simulink model "RC_Circuit_N16C_1"  (R2020b)
settings: Solver=VariableStepAuto  StartTime=0.0  StopTime=10.0  RelTol=1e-3
model workspace (MAT data in the model file):
  Cp = 1.49336e-12
  Cs = 9.6952e-12
  L = 1.154625e-06
  R = 24.7254
libraries: powerlib x51
settings Model: OrderedModelArguments=off  Creator=25085  LastModifiedBy=zq001
settings DebuggingCC: UnconnectedLineMsg=none

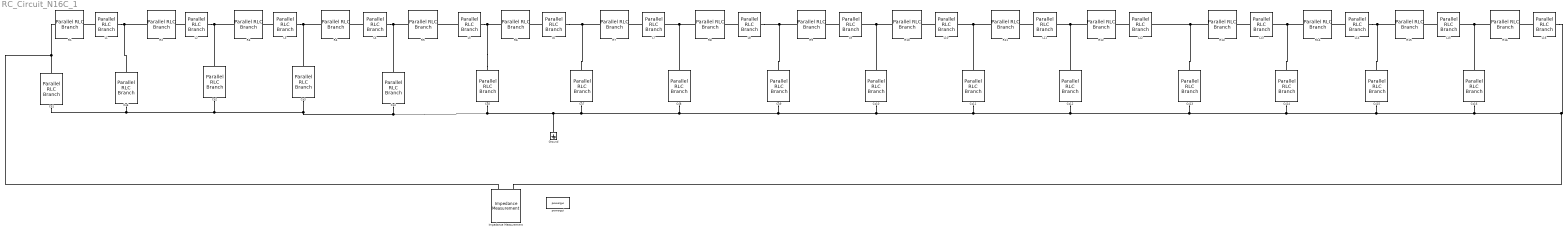
== system RC_Circuit_N16C_1 ==
  Cs{1..16} (16 alike) : powerlib/Elements/Parallel RLC Branch  LConnTagsString=a  RConnTagsString=__new0  BranchType=C  Resistance=1  Inductance=1e-3  SetiL0=off  InitialCurrent=0  Capacitance=Cs  Setx0=off  InitialVoltage=0  Measurements=None
  Ground : powerlib/Elements/Ground  LConnTagsString=a
  Impedance Measurement : powerlib/Measurements/Impedance Measurement  LConnTagsString=+|-  Factor=1
      settings: SourceProductBaseCode=PS
  L{1..16} (16 alike) : powerlib/Elements/Parallel RLC Branch  LConnTagsString=a  RConnTagsString=__new0  BranchType=L  Resistance=1  Inductance=L  SetiL0=off  InitialCurrent=0  Capacitance=1e-6  Setx0=off  InitialVoltage=0  Measurements=None
  R{1..16} (16 alike) : powerlib/Elements/Parallel RLC Branch  LConnTagsString=a  RConnTagsString=__new0  BranchType=R  Resistance=R  Inductance=1e-3  SetiL0=off  InitialCurrent=0  Capacitance=1e-6  Setx0=off  InitialVoltage=0  Measurements=None
  powergui : powerlib/powergui  Priority=1  SimulationMode=Continuous  SampleTime=50e-6  frequency=60  Iterations=50  frequencyindice=60  Pbase=100e6  ErrMax=1e-4  UnitsV=kV  UnitsW=MW  buscounter=0  FunctionMessages=off  echomessages=off  EnableUseOfTLC=off  CurrentSourceSwitches=off  DisableSnubberDevices=off  DisableRonSwitches=off  DisableVfSwitches=off  DisplayEquations=off  AutomaticDiscreteSolvers=off  SolverType=Tustin/Backward Euler (TBE)  Interpol=off  ExternalGateDelay=off  methode=off  Ts=100  x0status=blocks  SPID=on  SwTol=0  HookPort=off  NonlinearTolerance=1e-4  nMaxIteration=100  ContinueOnMaxIteration=off  RestoreLinks=warning  ResistiveCurrentMeasurement=off  Frange=[0:2:500]  Ylog=off  Xlog=on  ShowGrid=off  save=off  variable=ZData  structure=0  ZoomFFT=off  StartTime=0.0  cycles=1  DisplayStyle=1  fundamental=60  FreqAxis=off  MaxFrequency=1000  frequencyindicesteady=1  RmsSteady=1  display=off
  connections:
  L1/LConn1 -- R1/RConn1
  L2/LConn1 -- R2/RConn1
  Cs9/LConn1 -- L8/RConn1 -- R9/LConn1
  L3/LConn1 -- R3/RConn1
  L4/LConn1 -- R4/RConn1
  L6/LConn1 -- R6/RConn1
  L5/LConn1 -- R5/RConn1
  L7/LConn1 -- R7/RConn1
  Cs5/LConn1 -- R6/LConn1 -- L5/RConn1
  R5/LConn1 -- Cs4/LConn1 -- L4/RConn1
  Cs6/LConn1 -- L1/RConn1 -- R2/LConn1
  L3/RConn1 -- Cs3/LConn1 -- R4/LConn1
  R3/LConn1 -- Cs2/LConn1 -- L2/RConn1
  Impedance Measurement/LConn1 -- Cs1/LConn1 -- R1/LConn1
  Cs7/LConn1 -- R7/LConn1 -- L6/RConn1
  Cs8/LConn1 -- R8/LConn1 -- L7/RConn1
  L8/LConn1 -- R8/RConn1
  R10/LConn1 -- Cs10/LConn1 -- L9/RConn1
  L10/LConn1 -- R10/RConn1
  L9/LConn1 -- R9/RConn1
  Cs11/LConn1 -- R11/LConn1 -- L10/RConn1
  R12/LConn1 -- Cs12/LConn1 -- L11/RConn1
  L12/LConn1 -- R12/RConn1
  L11/LConn1 -- R11/RConn1
  Cs15/LConn1 -- L14/RConn1 -- R15/LConn1
  R14/LConn1 -- Cs14/LConn1 -- L13/RConn1
  L14/LConn1 -- R14/RConn1
  L13/LConn1 -- R13/RConn1
  R13/LConn1 -- Cs13/LConn1 -- L12/RConn1
  R16/LConn1 -- Cs16/LConn1 -- L15/RConn1
  L16/LConn1 -- R16/RConn1
  L15/LConn1 -- R15/RConn1
  Cs15/RConn1 -- Impedance Measurement/LConn2 -- L16/RConn1 -- Cs16/RConn1 -- Cs5/RConn1 -- Cs4/RConn1 -- Cs3/RConn1 -- Cs2/RConn1 -- Cs6/RConn1 -- Cs1/RConn1 -- Ground/LConn1 -- Cs7/RConn1 -- Cs8/RConn1 -- Cs9/RConn1 -- Cs10/RConn1 -- Cs11/RConn1 -- Cs12/RConn1 -- Cs13/RConn1 -- Cs14/RConn1
